simulink model "KE88_control"  (R2026a)
settings: Solver=VariableStepAuto
InitFcn:
  | KE88_parametros
undefined symbols (not defined in the file or in its folder): KE88_lee_mando

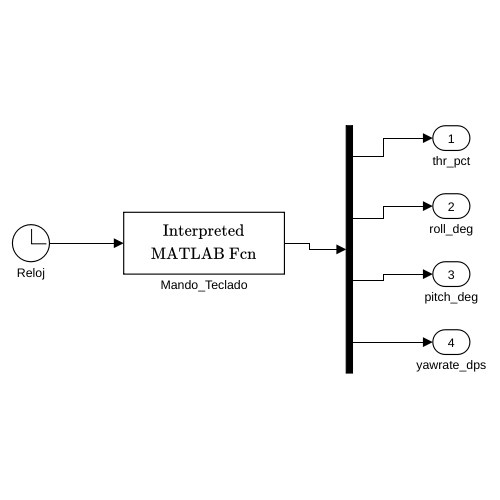
[thumbnail: Simulink's stored preview of the top-level diagram]
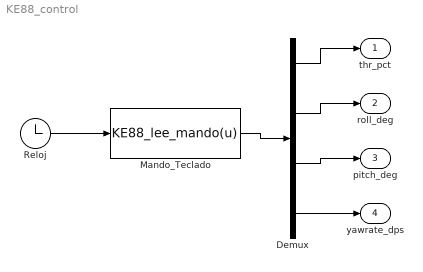
== system KE88_control ==
  Demux : Demux
  Mando_Teclado : MATLABFcn  MATLABFcn=KE88_lee_mando(u)  OutputDimensions=4
  Reloj : Clock
  thr_pct : Outport
  roll_deg : Outport  Port=2
  pitch_deg : Outport  Port=3
  yawrate_dps : Outport  Port=4
  wires:
  Reloj/1 -> Mando_Teclado/1
  Mando_Teclado/1 -> Demux/1
  Demux/1 -> thr_pct/1
  Demux/2 -> roll_deg/1
  Demux/3 -> pitch_deg/1
  Demux/4 -> yawrate_dps/1
